simulink model "modele_non_lineaire"  (R2016a)
settings: Solver=ode45  StartTime=0.0  StopTime=tfin  FixedStep=0.001  RelTol=1e-09
undefined symbols (not defined in the file or in its folder): ae0, ae1, ae2, ae3, as0, as1, as2, as3, Axeq, Ayeq, be1, g, ia_e, ib_e, ic_e, JS, Jx, LA, mP, mS, Pzeq, RA, rS, vx_s_e, vy_s_e, vz_e, w_phi_e, w_theta_e, XA, XB, XC, XD, XE, XF, xSeq, YA, YB, YC, YD, YE, YF, ySeq
settings Model: Creator=delafontaine  LastModifiedBy=theh2203
settings SolverCC: AlgebraicLoopSolver=LineSearch
settings DataIOCC: LimitDataPoints=on  SaveFormat=Array  SignalLoggingSaveFormat=ModelDataLogs
settings DebuggingCC: UnderspecifiedInitializationDetection=Classic  MergeDetectMultiDrivingBlocksExec=none  MultiTaskDSMMsg=warning  MultiTaskCondExecSysMsg=none
settings HardwareCC: ProdBitPerPointer=32  ProdLargestAtomicFloat=None  ProdIntDivRoundTo=Undefined  ProdEndianess=Unspecified  ProdWordSize=32  ProdHWDeviceType=32-bit Generic
settings ModelReferenceCC: PropagateSignalLabelsOutOfModel=off
settings ConfigComp: CovModelRefEnable=Off  CovSFcnEnable=off

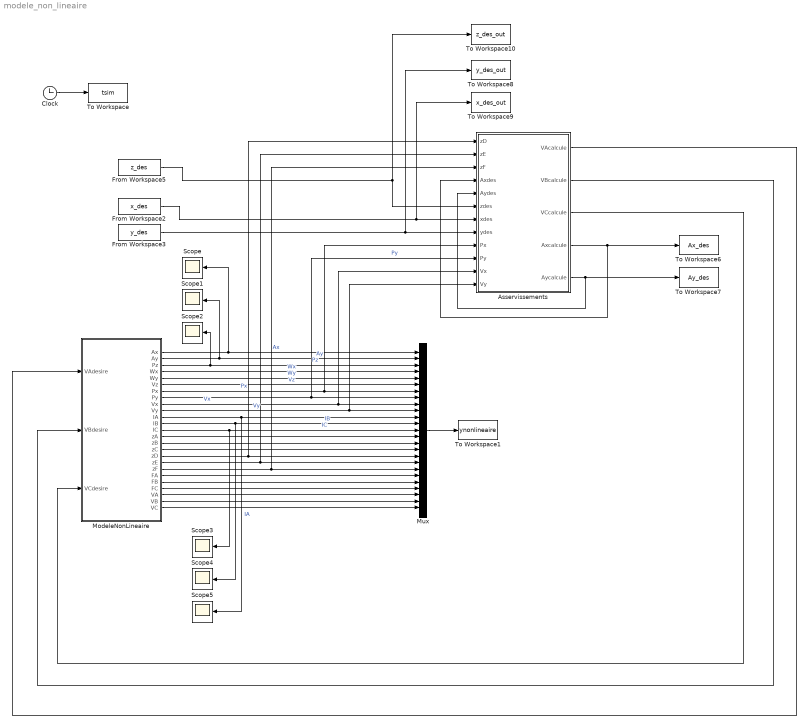
== system modele_non_lineaire ==
  Asservissements : Subsystem
      mask help: Simulink:masks:GenSFuncDesc_MD
      mask Help: eval('feval(''rtwprivate'',''rtwhelpview'',''rtw_sfcn_block'')');
  Clock : Clock
  From Workspace2 : FromWorkspace  VariableName=x_des  SampleTime=0  Interpolate=off  OutputAfterFinalValue=Holding final value
  From Workspace3 : FromWorkspace  VariableName=y_des  SampleTime=0  Interpolate=off  OutputAfterFinalValue=Holding final value
  From Workspace5 : FromWorkspace  VariableName=z_des  SampleTime=0  Interpolate=off  OutputAfterFinalValue=Holding final value
  ModeleNonLineaire : Subsystem
      mask help: Simulink:masks:GenSFuncDesc_MD
      mask Help: eval('feval(''rtwprivate'',''rtwhelpview'',''rtw_sfcn_block'')');
  Mux : Mux  Inputs=25
  Scope{,1..5} (6 alike) : Scope
  To Workspace : ToWorkspace  VariableName=tsim  SampleTime=-1
  To Workspace1 : ToWorkspace  VariableName=ynonlineaire  SampleTime=-1
  To Workspace10 : ToWorkspace  VariableName=z_des_out  SampleTime=-1
  To Workspace6 : ToWorkspace  VariableName=Ax_des  SampleTime=-1
  To Workspace7 : ToWorkspace  VariableName=Ay_des  SampleTime=-1
  To Workspace8 : ToWorkspace  VariableName=y_des_out  SampleTime=-1
  To Workspace9 : ToWorkspace  VariableName=x_des_out  SampleTime=-1
  wires:
  Mux/1 -> To Workspace1/1
  Clock/1 -> To Workspace/1
  From Workspace5/1 -> Asservissements/6(zdes), To Workspace10/1
  ModeleNonLineaire/1(Ax) -> Scope/1, Mux/1  "Ax"
  ModeleNonLineaire/2(Ay) -> Scope1/1, Mux/2  "Ay"
  ModeleNonLineaire/3(Pz) -> Scope2/1, Mux/3  "Pz"
  ModeleNonLineaire/4(Wx) -> Mux/4  "Wx"
  ModeleNonLineaire/5(Wy) -> Mux/5  "Wy"
  ModeleNonLineaire/6(Vz) -> Mux/6  "Vz"
  ModeleNonLineaire/7(Px) -> Asservissements/9(Px), Mux/7  "Px"
  ModeleNonLineaire/8(Py) -> Asservissements/10(Py), Mux/8  "Py"
  ModeleNonLineaire/9(Vx) -> Asservissements/11(Vx), Mux/9  "Vx"
  ModeleNonLineaire/10(Vy) -> Asservissements/12(Vy), Mux/10  "Vy"
  ModeleNonLineaire/11(IA) -> Scope5/1, Mux/11  "IA"
  ModeleNonLineaire/12(IB) -> Scope4/1, Mux/12  "IB"
  ModeleNonLineaire/13(IC) -> Scope3/1, Mux/13  "IC"
  From Workspace3/1 -> Asservissements/8(ydes), To Workspace8/1
  From Workspace2/1 -> Asservissements/7(xdes), To Workspace9/1
  ModeleNonLineaire/20(FA) -> Mux/20
  ModeleNonLineaire/21(FB) -> Mux/21
  ModeleNonLineaire/22(FC) -> Mux/22
  ModeleNonLineaire/23(VA) -> Mux/23
  ModeleNonLineaire/24(VB) -> Mux/24
  ModeleNonLineaire/25(VC) -> Mux/25
  ModeleNonLineaire/17(zD) -> Asservissements/1(zD), Mux/17
  ModeleNonLineaire/18(zE) -> Mux/18, Asservissements/2(zE)
  ModeleNonLineaire/19(zF) -> Asservissements/3(zF), Mux/19
  ModeleNonLineaire/14(zA) -> Mux/14
  ModeleNonLineaire/16(zC) -> Mux/16
  Asservissements/4(Axcalcule) -> Asservissements/4(Axdes), To Workspace6/1
  Asservissements/5(Aycalcule) -> Asservissements/5(Aydes), To Workspace7/1
  Asservissements/1(VAcalcule) -> ModeleNonLineaire/1(VAdesire)
  Asservissements/2(VBcalcule) -> ModeleNonLineaire/2(VBdesire)
  Asservissements/3(VCcalcule) -> ModeleNonLineaire/3(VCdesire)
  ModeleNonLineaire/15(zB) -> Mux/15

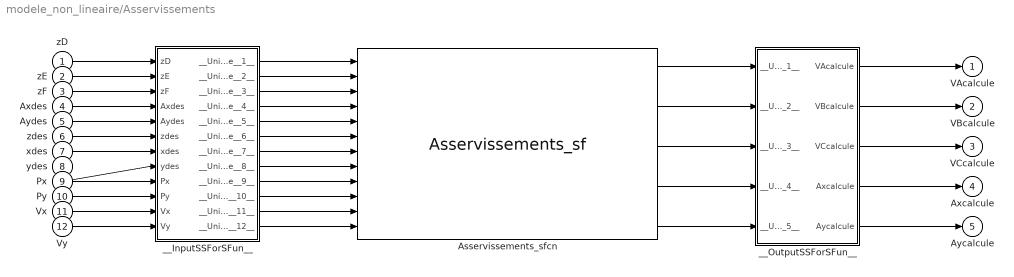
== system modele_non_lineaire/Asservissements ==
  zD : Inport
  zE : Inport  Port=2
  zF : Inport  Port=3
  Axdes : Inport  Port=4
  Aydes : Inport  Port=5
  zdes : Inport  Port=6
  xdes : Inport  Port=7
  ydes : Inport  Port=8
  Px : Inport  Port=9
  Py : Inport  Port=10
  Vx : Inport  Port=11
  Vy : Inport  Port=12
  Asservissements_sfcn : S-Function  FunctionName=Asservissements_sf  SFunctionModules=""  SFunctionDeploymentMode=off  EnableBusSupport=off  mask{rtw_sf_name=Asservissements_sf, showVar=off}
      mask prompts: rtw_sf_name "Simulink:masks:GenSFuncName_MP"; showVar "Simulink:masks:GenSFuncShowModuleList_MP"
      mask help: Simulink:masks:GenSFuncDesc_MD
      mask init:
      | displist = '';
      | if ~strcmp(get_param(gcb, 'FunctionName'), rtw_sf_name);
      |   set_param(gcb, 'FunctionName', rtw_sf_name);
      | end
      | % Check if we are generating code
      | rtw_mode = false;
      | if strcmpi(get_param(bdroot(gcb),'SimulationStatus'),'Initializing')
      | 	rtw_mode = strcmpi(get_param(bdroot(gcb),'BuildingRTWCode'),'on') && ...
      | 		~strcmpi(get_param(bdroot(gcb),'TargetStyle'),'SimulationTarget');
      | end
      | if showVar || rtw_mode
      | 	if exist('rtwsfunc') == 2 | exist('rtwsfunc') == 6
      | 		tmplist = rtwsfunc(rtw_sf_name,gcb);
      | 		tmplist = DAStudio.message('Simulink:masks:GenSFuncListOfModules_IC', tmplist);
      | 	elseif showVar
      | 		tmplist1 = DAStudio.message('Simulink:masks:GenSFuncListOfModules_IC', '');
      |         tmplist2 = DAStudio.message('Simulink:masks:GenSFuncNotLicensed_IC');
      |         tmplist = [tmplist1 tmplist2];
      |  	end
      | end
      | if showVar
      |   displist = tmplist;
      | end
      settings: CopyFcn=|
      | if ~strcmp(get_param(gcb,'Linkstatus'),'none') && ...
      | ~strcmp(get_param(gcb,'Linkstatus'),'implicit')
      |   set_param(gcb,'LinkStatus','none');
      | end
      mask Help: eval('feval(''rtwprivate'',''rtwhelpview'',''rtw_sfcn_block'')');
      mask Display:
      | port_label('input',1,'zD');
      | port_label('input',2,'zE');
      | port_label('input',3,'zF');
      | port_label('input',4,'Axdes');
      | port_label('input',5,'Aydes');
      | port_label('input',6,'zdes');
      | port_label('input',7,'xdes');
      | port_label('input',8,'ydes');
      | port_label('input',9,'Px');
      | port_label('input',10,'Py');
      | port_label('input',11,'Vx');
      | port_label('input',12,'Vy');
      | port_label('output',1,'VAcalcule');
      | port_label('output',2,'VBcalcule');
      | port_label('output',3,'VCcalcule');
      | port_label('output',4,'Axcalcule');
      | port_label('output',5,'Aycalcule');
  __InputSSForSFun__ : Subsystem
  __OutputSSForSFun__ : Subsystem
  VAcalcule : Outport
  VBcalcule : Outport  Port=2
  VCcalcule : Outport  Port=3
  Axcalcule : Outport  Port=4
  Aycalcule : Outport  Port=5
  wires:
  zD/1 -> __InputSSForSFun__/1(zD)
  zE/1 -> __InputSSForSFun__/2(zE)
  zF/1 -> __InputSSForSFun__/3(zF)
  Axdes/1 -> __InputSSForSFun__/4(Axdes)
  Aydes/1 -> __InputSSForSFun__/5(Aydes)
  zdes/1 -> __InputSSForSFun__/6(zdes)
  xdes/1 -> __InputSSForSFun__/7(xdes)
  ydes/1 -> __InputSSForSFun__/8(ydes)
  Px/1 -> __InputSSForSFun__/9(Px)
  Py/1 -> __InputSSForSFun__/10(Py)
  Vx/1 -> __InputSSForSFun__/11(Vx)
  Vy/1 -> __InputSSForSFun__/12(Vy)
  __InputSSForSFun__/1(__UniqueOutportName__1__) -> Asservissements_sfcn/1
  __InputSSForSFun__/2(__UniqueOutportName__2__) -> Asservissements_sfcn/2
  __InputSSForSFun__/3(__UniqueOutportName__3__) -> Asservissements_sfcn/3
  __InputSSForSFun__/4(__UniqueOutportName__4__) -> Asservissements_sfcn/4
  __InputSSForSFun__/5(__UniqueOutportName__5__) -> Asservissements_sfcn/5
  __InputSSForSFun__/6(__UniqueOutportName__6__) -> Asservissements_sfcn/6
  __InputSSForSFun__/7(__UniqueOutportName__7__) -> Asservissements_sfcn/7
  __InputSSForSFun__/8(__UniqueOutportName__8__) -> Asservissements_sfcn/8
  __InputSSForSFun__/9(__UniqueOutportName__9__) -> Asservissements_sfcn/9
  __InputSSForSFun__/10(__UniqueOutportName__10__) -> Asservissements_sfcn/10
  __InputSSForSFun__/11(__UniqueOutportName__11__) -> Asservissements_sfcn/11
  __InputSSForSFun__/12(__UniqueOutportName__12__) -> Asservissements_sfcn/12
  Asservissements_sfcn/1 -> __OutputSSForSFun__/1(__UniqueInportName__1__)
  Asservissements_sfcn/2 -> __OutputSSForSFun__/2(__UniqueInportName__2__)
  Asservissements_sfcn/3 -> __OutputSSForSFun__/3(__UniqueInportName__3__)
  Asservissements_sfcn/4 -> __OutputSSForSFun__/4(__UniqueInportName__4__)
  Asservissements_sfcn/5 -> __OutputSSForSFun__/5(__UniqueInportName__5__)
  __OutputSSForSFun__/1(VAcalcule) -> VAcalcule/1
  __OutputSSForSFun__/2(VBcalcule) -> VBcalcule/1
  __OutputSSForSFun__/3(VCcalcule) -> VCcalcule/1
  __OutputSSForSFun__/4(Axcalcule) -> Axcalcule/1
  __OutputSSForSFun__/5(Aycalcule) -> Aycalcule/1

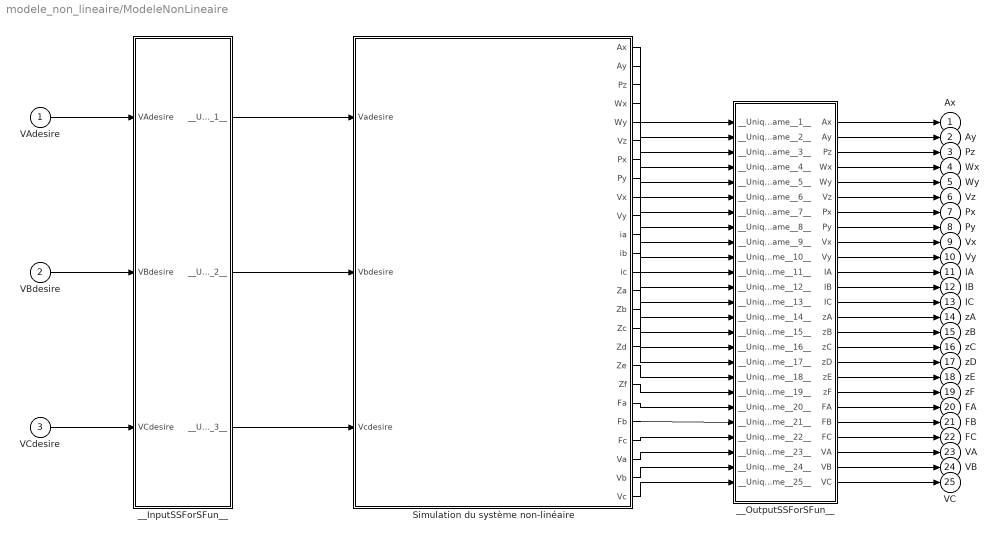
== system modele_non_lineaire/ModeleNonLineaire ==
  VAdesire : Inport
  VBdesire : Inport  Port=2
  VCdesire : Inport  Port=3
  Simulation du système non-linéaire : Subsystem
  __InputSSForSFun__ : Subsystem
  __OutputSSForSFun__ : Subsystem
  Ax : Outport
  Ay : Outport  Port=2
  Pz : Outport  Port=3
  Wx : Outport  Port=4
  Wy : Outport  Port=5
  Vz : Outport  Port=6
  Px : Outport  Port=7
  Py : Outport  Port=8
  Vx : Outport  Port=9
  Vy : Outport  Port=10
  IA : Outport  Port=11
  IB : Outport  Port=12
  IC : Outport  Port=13
  zA : Outport  Port=14
  zB : Outport  Port=15
  zC : Outport  Port=16
  zD : Outport  Port=17
  zE : Outport  Port=18
  zF : Outport  Port=19
  FA : Outport  Port=20
  FB : Outport  Port=21
  FC : Outport  Port=22
  VA : Outport  Port=23
  VB : Outport  Port=24
  VC : Outport  Port=25
  wires:
  VAdesire/1 -> __InputSSForSFun__/1(VAdesire)
  VBdesire/1 -> __InputSSForSFun__/2(VBdesire)
  VCdesire/1 -> __InputSSForSFun__/3(VCdesire)
  __InputSSForSFun__/1(__UniqueOutportName__1__) -> Simulation du système non-linéaire/1(Vadesire)
  __InputSSForSFun__/2(__UniqueOutportName__2__) -> Simulation du système non-linéaire/2(Vbdesire)
  __InputSSForSFun__/3(__UniqueOutportName__3__) -> Simulation du système non-linéaire/3(Vcdesire)
  Simulation du système non-linéaire/1(Ax) -> __OutputSSForSFun__/1(__UniqueInportName__1__)
  Simulation du système non-linéaire/2(Ay) -> __OutputSSForSFun__/2(__UniqueInportName__2__)
  Simulation du système non-linéaire/3(Pz) -> __OutputSSForSFun__/3(__UniqueInportName__3__)
  Simulation du système non-linéaire/4(Wx) -> __OutputSSForSFun__/4(__UniqueInportName__4__)
  Simulation du système non-linéaire/5(Wy) -> __OutputSSForSFun__/5(__UniqueInportName__5__)
  Simulation du système non-linéaire/6(Vz) -> __OutputSSForSFun__/6(__UniqueInportName__6__)
  Simulation du système non-linéaire/7(Px) -> __OutputSSForSFun__/7(__UniqueInportName__7__)
  Simulation du système non-linéaire/8(Py) -> __OutputSSForSFun__/8(__UniqueInportName__8__)
  Simulation du système non-linéaire/9(Vx) -> __OutputSSForSFun__/9(__UniqueInportName__9__)
  Simulation du système non-linéaire/10(Vy) -> __OutputSSForSFun__/10(__UniqueInportName__10__)
  Simulation du système non-linéaire/11(ia) -> __OutputSSForSFun__/11(__UniqueInportName__11__)
  Simulation du système non-linéaire/12(ib) -> __OutputSSForSFun__/12(__UniqueInportName__12__)
  Simulation du système non-linéaire/13(ic) -> __OutputSSForSFun__/13(__UniqueInportName__13__)
  Simulation du système non-linéaire/14(Za) -> __OutputSSForSFun__/14(__UniqueInportName__14__)
  Simulation du système non-linéaire/15(Zb) -> __OutputSSForSFun__/15(__UniqueInportName__15__)
  Simulation du système non-linéaire/16(Zc) -> __OutputSSForSFun__/16(__UniqueInportName__16__)
  Simulation du système non-linéaire/17(Zd) -> __OutputSSForSFun__/17(__UniqueInportName__17__)
  Simulation du système non-linéaire/18(Ze) -> __OutputSSForSFun__/18(__UniqueInportName__18__)
  Simulation du système non-linéaire/19(Zf) -> __OutputSSForSFun__/19(__UniqueInportName__19__)
  Simulation du système non-linéaire/20(Fa) -> __OutputSSForSFun__/20(__UniqueInportName__20__)
  Simulation du système non-linéaire/21(Fb) -> __OutputSSForSFun__/21(__UniqueInportName__21__)
  Simulation du système non-linéaire/22(Fc) -> __OutputSSForSFun__/22(__UniqueInportName__22__)
  Simulation du système non-linéaire/23(Va) -> __OutputSSForSFun__/23(__UniqueInportName__23__)
  Simulation du système non-linéaire/24(Vb) -> __OutputSSForSFun__/24(__UniqueInportName__24__)
  Simulation du système non-linéaire/25(Vc) -> __OutputSSForSFun__/25(__UniqueInportName__25__)
  __OutputSSForSFun__/1(Ax) -> Ax/1
  __OutputSSForSFun__/2(Ay) -> Ay/1
  __OutputSSForSFun__/3(Pz) -> Pz/1
  __OutputSSForSFun__/4(Wx) -> Wx/1
  __OutputSSForSFun__/5(Wy) -> Wy/1
  __OutputSSForSFun__/6(Vz) -> Vz/1
  __OutputSSForSFun__/7(Px) -> Px/1
  __OutputSSForSFun__/8(Py) -> Py/1
  __OutputSSForSFun__/9(Vx) -> Vx/1
  __OutputSSForSFun__/10(Vy) -> Vy/1
  __OutputSSForSFun__/11(IA) -> IA/1
  __OutputSSForSFun__/12(IB) -> IB/1
  __OutputSSForSFun__/13(IC) -> IC/1
  __OutputSSForSFun__/14(zA) -> zA/1
  __OutputSSForSFun__/15(zB) -> zB/1
  __OutputSSForSFun__/16(zC) -> zC/1
  __OutputSSForSFun__/17(zD) -> zD/1
  __OutputSSForSFun__/18(zE) -> zE/1
  __OutputSSForSFun__/19(zF) -> zF/1
  __OutputSSForSFun__/20(FA) -> FA/1
  __OutputSSForSFun__/21(FB) -> FB/1
  __OutputSSForSFun__/22(FC) -> FC/1
  __OutputSSForSFun__/23(VA) -> VA/1
  __OutputSSForSFun__/24(VB) -> VB/1
  __OutputSSForSFun__/25(VC) -> VC/1

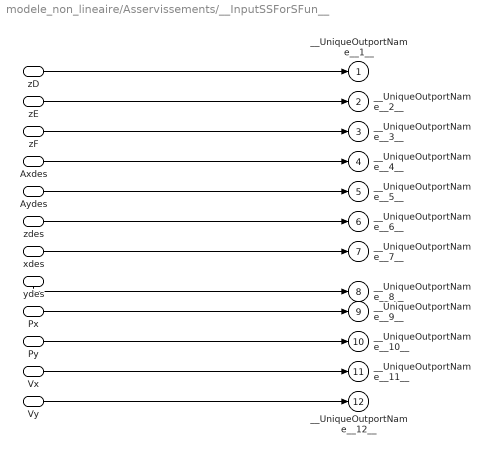
== system modele_non_lineaire/Asservissements/__InputSSForSFun__ ==
  zD : Inport
  zE : Inport  Port=2
  zF : Inport  Port=3
  Axdes : Inport  Port=4
  Aydes : Inport  Port=5
  zdes : Inport  Port=6
  xdes : Inport  Port=7
  ydes : Inport  Port=8
  Px : Inport  Port=9
  Py : Inport  Port=10
  Vx : Inport  Port=11
  Vy : Inport  Port=12
  __UniqueOutportName__1__ : Outport
  __UniqueOutportName__2__ : Outport  Port=2
  __UniqueOutportName__3__ : Outport  Port=3
  __UniqueOutportName__4__ : Outport  Port=4
  __UniqueOutportName__5__ : Outport  Port=5
  __UniqueOutportName__6__ : Outport  Port=6
  __UniqueOutportName__7__ : Outport  Port=7
  __UniqueOutportName__8__ : Outport  Port=8
  __UniqueOutportName__9__ : Outport  Port=9
  __UniqueOutportName__10__ : Outport  Port=10
  __UniqueOutportName__11__ : Outport  Port=11
  __UniqueOutportName__12__ : Outport  Port=12
  wires:
  zD/1 -> __UniqueOutportName__1__/1
  zE/1 -> __UniqueOutportName__2__/1
  zF/1 -> __UniqueOutportName__3__/1
  Axdes/1 -> __UniqueOutportName__4__/1
  Aydes/1 -> __UniqueOutportName__5__/1
  zdes/1 -> __UniqueOutportName__6__/1
  xdes/1 -> __UniqueOutportName__7__/1
  ydes/1 -> __UniqueOutportName__8__/1
  Px/1 -> __UniqueOutportName__9__/1
  Py/1 -> __UniqueOutportName__10__/1
  Vx/1 -> __UniqueOutportName__11__/1
  Vy/1 -> __UniqueOutportName__12__/1

== system modele_non_lineaire/Asservissements/__OutputSSForSFun__ ==
  __UniqueInportName__1__ : Inport
  __UniqueInportName__2__ : Inport  Port=2
  __UniqueInportName__3__ : Inport  Port=3
  __UniqueInportName__4__ : Inport  Port=4
  __UniqueInportName__5__ : Inport  Port=5
  VAcalcule : Outport
  VBcalcule : Outport  Port=2
  VCcalcule : Outport  Port=3
  Axcalcule : Outport  Port=4
  Aycalcule : Outport  Port=5
  wires:
  __UniqueInportName__1__/1 -> VAcalcule/1
  __UniqueInportName__2__/1 -> VBcalcule/1
  __UniqueInportName__3__/1 -> VCcalcule/1
  __UniqueInportName__4__/1 -> Axcalcule/1  "Ax_des"
  __UniqueInportName__5__/1 -> Aycalcule/1  "Ay_des"

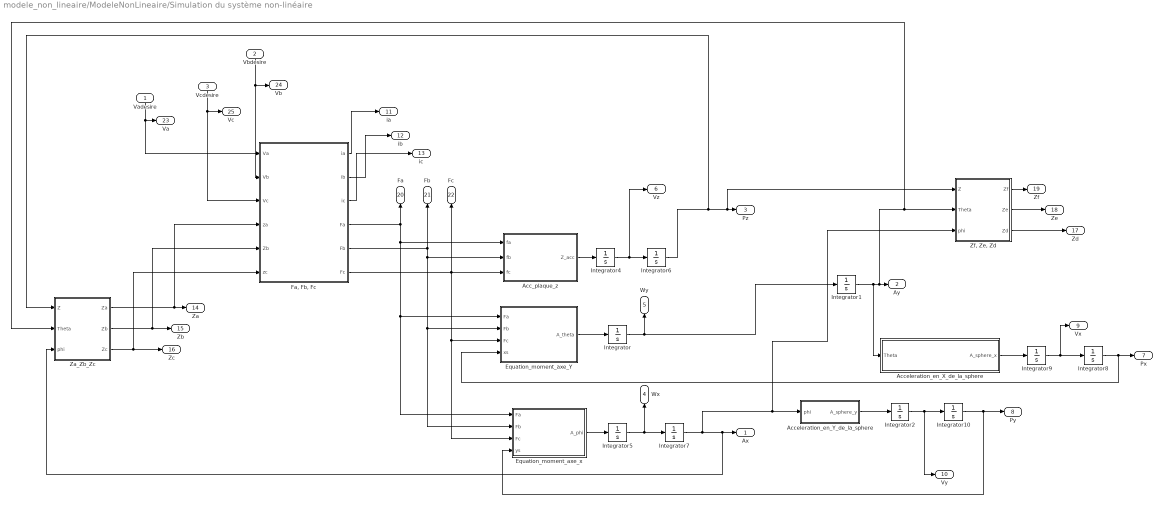
== system modele_non_lineaire/ModeleNonLineaire/Simulation du système non-linéaire ==
  Vadesire : Inport
  Vbdesire : Inport  Port=2
  Vcdesire : Inport  Port=3
  Acc_plaque_z : Subsystem
  Acceleration_en_X_de_la_sphere : Subsystem
  Acceleration_en_Y_de_la_sphere : Subsystem
  Equation_moment_axe_Y : Subsystem
  Equation_moment_axe_x : Subsystem
  "Fa, Fb, Fc" : Subsystem
  Integrator : Integrator  InitialCondition=w_theta_e
  Integrator1 : Integrator  InitialCondition=Ayeq
  Integrator10 : Integrator  InitialCondition=ySeq
  Integrator2 : Integrator  InitialCondition=vy_s_e
  Integrator4 : Integrator  InitialCondition=vz_e
  Integrator5 : Integrator  InitialCondition=w_phi_e
  Integrator6 : Integrator  InitialCondition=Pzeq
  Integrator7 : Integrator  InitialCondition=Axeq
  Integrator8 : Integrator  InitialCondition=xSeq
  Integrator9 : Integrator  InitialCondition=vx_s_e
  Za_Zb_Zc : Subsystem
  "Zf, Ze, Zd" : Subsystem
  Ax : Outport
  Ay : Outport  Port=2
  Pz : Outport  Port=3
  Wx : Outport  Port=4
  Wy : Outport  Port=5
  Vz : Outport  Port=6
  Px : Outport  Port=7
  Py : Outport  Port=8
  Vx : Outport  Port=9
  Vy : Outport  Port=10
  ia : Outport  Port=11
  ib : Outport  Port=12
  ic : Outport  Port=13
  Za : Outport  Port=14
  Zb : Outport  Port=15
  Zc : Outport  Port=16
  Zd : Outport  Port=17
  Ze : Outport  Port=18
  Zf : Outport  Port=19
  Fa : Outport  Port=20
  Fb : Outport  Port=21
  Fc : Outport  Port=22
  Va : Outport  Port=23
  Vb : Outport  Port=24
  Vc : Outport  Port=25
  wires:
  Vadesire/1 -> "Fa, Fb, Fc"/1(Va), Va/1
  "Fa, Fb, Fc"/3(ic) -> ic/1
  "Fa, Fb, Fc"/1(ia) -> ia/1
  "Fa, Fb, Fc"/2(ib) -> ib/1
  Vcdesire/1 -> "Fa, Fb, Fc"/3(Vc), Vc/1
  Vbdesire/1 -> Vb/1, "Fa, Fb, Fc"/2(Vb)
  "Zf, Ze, Zd"/1(Zf) -> Zf/1
  "Zf, Ze, Zd"/2(Ze) -> Ze/1
  "Zf, Ze, Zd"/3(Zd) -> Zd/1
  Integrator/1 -> Integrator1/1, Wy/1
  Integrator1/1 -> Acceleration_en_X_de_la_sphere/1(Theta), Za_Zb_Zc/2(Theta), "Zf, Ze, Zd"/2(Theta), Ay/1
  Integrator5/1 -> Integrator7/1, Wx/1
  Integrator7/1 -> "Zf, Ze, Zd"/3(phi), Acceleration_en_Y_de_la_sphere/1(phi), Za_Zb_Zc/3(phi), Ax/1
  Acc_plaque_z/1(Z_acc) -> Integrator4/1
  Integrator4/1 -> Vz/1, Integrator6/1
  Integrator6/1 -> Za_Zb_Zc/1(Z), "Zf, Ze, Zd"/1(Z), Pz/1
  Acceleration_en_X_de_la_sphere/1(A_sphere_x) -> Integrator9/1
  Integrator9/1 -> Vx/1, Integrator8/1
  Integrator8/1 -> Equation_moment_axe_Y/4(xs), Px/1
  Integrator10/1 -> Equation_moment_axe_x/4(ys), Py/1
  Acceleration_en_Y_de_la_sphere/1(A_sphere_y) -> Integrator2/1
  Integrator2/1 -> Vy/1, Integrator10/1
  Za_Zb_Zc/1(Za) -> "Fa, Fb, Fc"/4(za), Za/1
  Za_Zb_Zc/2("Zb ") -> "Fa, Fb, Fc"/5(Zb), Zb/1
  Za_Zb_Zc/3(Zc) -> "Fa, Fb, Fc"/6(zc), Zc/1
  Equation_moment_axe_x/1(A_phi) -> Integrator5/1
  Equation_moment_axe_Y/1(A_theta) -> Integrator/1
  "Fa, Fb, Fc"/4(Fa) -> Fa/1, Equation_moment_axe_x/1(Fa), Equation_moment_axe_Y/1(Fa), Acc_plaque_z/1(fa)
  "Fa, Fb, Fc"/5(Fb) -> Fb/1, Equation_moment_axe_x/2(Fb), Equation_moment_axe_Y/2(Fb), Acc_plaque_z/2(fb)
  "Fa, Fb, Fc"/6(Fc) -> Equation_moment_axe_x/3(Fc), Equation_moment_axe_Y/3(Fc), Fc/1, Acc_plaque_z/3(fc)

== system modele_non_lineaire/ModeleNonLineaire/__InputSSForSFun__ ==
  VAdesire : Inport
  VBdesire : Inport  Port=2
  VCdesire : Inport  Port=3
  __UniqueOutportName__1__ : Outport
  __UniqueOutportName__2__ : Outport  Port=2
  __UniqueOutportName__3__ : Outport  Port=3
  wires:
  VAdesire/1 -> __UniqueOutportName__1__/1
  VBdesire/1 -> __UniqueOutportName__2__/1
  VCdesire/1 -> __UniqueOutportName__3__/1

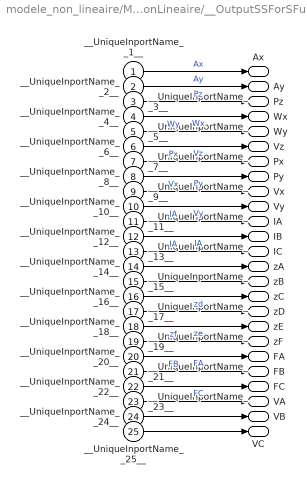
== system modele_non_lineaire/ModeleNonLineaire/__OutputSSForSFun__ ==
  __UniqueInportName__1__ : Inport
  __UniqueInportName__2__ : Inport  Port=2
  __UniqueInportName__3__ : Inport  Port=3
  __UniqueInportName__4__ : Inport  Port=4
  __UniqueInportName__5__ : Inport  Port=5
  __UniqueInportName__6__ : Inport  Port=6
  __UniqueInportName__7__ : Inport  Port=7
  __UniqueInportName__8__ : Inport  Port=8
  __UniqueInportName__9__ : Inport  Port=9
  __UniqueInportName__10__ : Inport  Port=10
  __UniqueInportName__11__ : Inport  Port=11
  __UniqueInportName__12__ : Inport  Port=12
  __UniqueInportName__13__ : Inport  Port=13
  __UniqueInportName__14__ : Inport  Port=14
  __UniqueInportName__15__ : Inport  Port=15
  __UniqueInportName__16__ : Inport  Port=16
  __UniqueInportName__17__ : Inport  Port=17
  __UniqueInportName__18__ : Inport  Port=18
  __UniqueInportName__19__ : Inport  Port=19
  __UniqueInportName__20__ : Inport  Port=20
  __UniqueInportName__21__ : Inport  Port=21
  __UniqueInportName__22__ : Inport  Port=22
  __UniqueInportName__23__ : Inport  Port=23
  __UniqueInportName__24__ : Inport  Port=24
  __UniqueInportName__25__ : Inport  Port=25
  Ax : Outport
  Ay : Outport  Port=2
  Pz : Outport  Port=3
  Wx : Outport  Port=4
  Wy : Outport  Port=5
  Vz : Outport  Port=6
  Px : Outport  Port=7
  Py : Outport  Port=8
  Vx : Outport  Port=9
  Vy : Outport  Port=10
  IA : Outport  Port=11
  IB : Outport  Port=12
  IC : Outport  Port=13
  zA : Outport  Port=14
  zB : Outport  Port=15
  zC : Outport  Port=16
  zD : Outport  Port=17
  zE : Outport  Port=18
  zF : Outport  Port=19
  FA : Outport  Port=20
  FB : Outport  Port=21
  FC : Outport  Port=22
  VA : Outport  Port=23
  VB : Outport  Port=24
  VC : Outport  Port=25
  wires:
  __UniqueInportName__1__/1 -> Ax/1  "Ax"
  __UniqueInportName__2__/1 -> Ay/1  "Ay"
  __UniqueInportName__3__/1 -> Pz/1  "Pz"
  __UniqueInportName__4__/1 -> Wx/1  "Wx"
  __UniqueInportName__5__/1 -> Wy/1  "Wy"
  __UniqueInportName__6__/1 -> Vz/1  "Vz"
  __UniqueInportName__7__/1 -> Px/1  "Px"
  __UniqueInportName__8__/1 -> Py/1  "Py"
  __UniqueInportName__9__/1 -> Vx/1  "Vx"
  __UniqueInportName__10__/1 -> Vy/1  "Vy"
  __UniqueInportName__11__/1 -> IA/1  "IA"
  __UniqueInportName__12__/1 -> IB/1  "IA"
  __UniqueInportName__13__/1 -> IC/1  "IA"
  __UniqueInportName__14__/1 -> zA/1
  __UniqueInportName__15__/1 -> zB/1
  __UniqueInportName__16__/1 -> zC/1
  __UniqueInportName__17__/1 -> zD/1  "zd"
  __UniqueInportName__18__/1 -> zE/1  "ze"
  __UniqueInportName__19__/1 -> zF/1  "zf"
  __UniqueInportName__20__/1 -> FA/1  "FA"
  __UniqueInportName__21__/1 -> FB/1  "FB"
  __UniqueInportName__22__/1 -> FC/1  "FC"
  __UniqueInportName__23__/1 -> VA/1
  __UniqueInportName__24__/1 -> VB/1
  __UniqueInportName__25__/1 -> VC/1

== system modele_non_lineaire/ModeleNonLineaire/Simulation du système non-linéaire/Acc_plaque_z ==
  fa : Inport
  fb : Inport  Port=2
  fc : Inport  Port=3
  Add : Sum  Inputs=++++
  Divide : Product  Inputs=*/
  Gain : Gain  Gain=g
  "masse_plaque-sphere " : Constant  Value=mP+mS
  Z_acc : Outport
  wires:
  fa/1 -> Add/1
  fc/1 -> Add/3
  fb/1 -> Add/2
  Add/1 -> Divide/1
  Divide/1 -> Z_acc/1
  "masse_plaque-sphere "/1 -> Divide/2, Gain/1
  Gain/1 -> Add/4

== system modele_non_lineaire/ModeleNonLineaire/Simulation du système non-linéaire/Acceleration_en_X_de_la_sphere ==
  Theta : Inport
  Add : Sum
  Constant : Constant  Value=mS
  Constant1 : Constant  Value=JS/rS^2
  Divide : Product  Inputs=*/
  Gain : Gain  Gain=-g*mS
  A_sphere_x : Outport
  wires:
  Theta/1 -> Gain/1
  Gain/1 -> Divide/1
  Constant1/1 -> Add/2
  Constant/1 -> Add/1
  Add/1 -> Divide/2
  Divide/1 -> A_sphere_x/1

== system modele_non_lineaire/ModeleNonLineaire/Simulation du système non-linéaire/Acceleration_en_Y_de_la_sphere ==
  phi : Inport
  Add : Sum
  Constant : Constant  Value=mS
  Constant1 : Constant  Value=JS/rS^2
  Divide : Product  Inputs=*/
  Gain : Gain  Gain=g*mS
  A_sphere_y : Outport
  wires:
  phi/1 -> Gain/1
  Gain/1 -> Divide/1
  Constant1/1 -> Add/2
  Constant/1 -> Add/1
  Add/1 -> Divide/2
  Divide/1 -> A_sphere_y/1

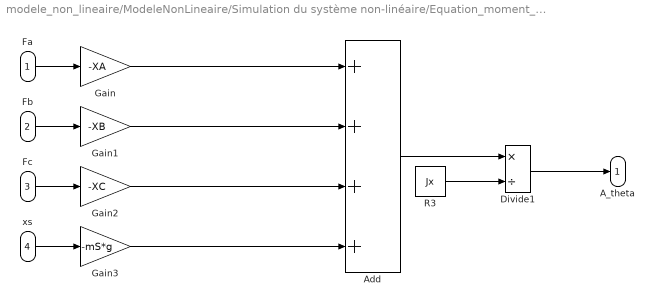
== system modele_non_lineaire/ModeleNonLineaire/Simulation du système non-linéaire/Equation_moment_axe_Y ==
  Fa : Inport
  Fb : Inport  Port=2
  Fc : Inport  Port=3
  xs : Inport  Port=4
  Add : Sum  Inputs=++++
  Divide1 : Product  Inputs=*/
  Gain : Gain  Gain=-XA
  Gain1 : Gain  Gain=-XB
  Gain2 : Gain  Gain=-XC
  Gain3 : Gain  Gain=-mS*g
  R3 : Constant  Value=Jx
  A_theta : Outport
  wires:
  Add/1 -> Divide1/1
  Divide1/1 -> A_theta/1
  Fa/1 -> Gain/1
  Gain/1 -> Add/1
  Fb/1 -> Gain1/1
  Fc/1 -> Gain2/1
  Gain2/1 -> Add/3
  Gain1/1 -> Add/2
  xs/1 -> Gain3/1
  R3/1 -> Divide1/2
  Gain3/1 -> Add/4

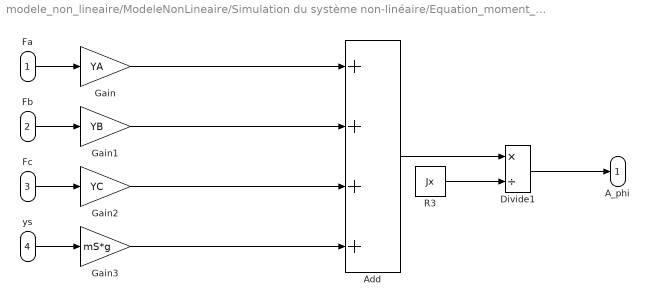
== system modele_non_lineaire/ModeleNonLineaire/Simulation du système non-linéaire/Equation_moment_axe_x ==
  Fa : Inport
  Fb : Inport  Port=2
  Fc : Inport  Port=3
  ys : Inport  Port=4
  Add : Sum  Inputs=++++
  Divide1 : Product  Inputs=*/
  Gain : Gain  Gain=YA
  Gain1 : Gain  Gain=YB
  Gain2 : Gain  Gain=YC
  Gain3 : Gain  Gain=mS*g
  R3 : Constant  Value=Jx
  A_phi : Outport
  wires:
  Gain3/1 -> Add/4
  R3/1 -> Divide1/2
  ys/1 -> Gain3/1
  Gain1/1 -> Add/2
  Gain2/1 -> Add/3
  Fc/1 -> Gain2/1
  Fb/1 -> Gain1/1
  Gain/1 -> Add/1
  Fa/1 -> Gain/1
  Divide1/1 -> A_phi/1
  Add/1 -> Divide1/1

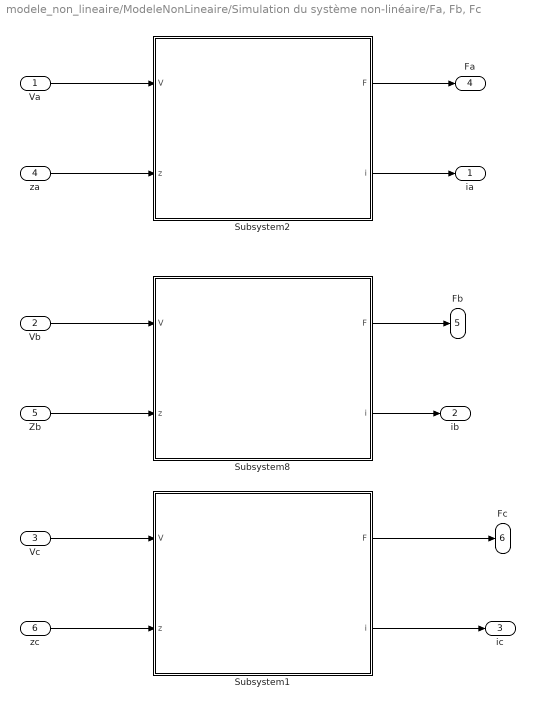
== system modele_non_lineaire/ModeleNonLineaire/Simulation du système non-linéaire/Fa, Fb, Fc ==
  Va : Inport
  Vb : Inport  Port=2
  Vc : Inport  Port=3
  za : Inport  Port=4
  Zb : Inport  Port=5
  zc : Inport  Port=6
  Subsystem1 : Subsystem
  Subsystem2 : Subsystem
  Subsystem8 : Subsystem
  ia : Outport
  ib : Outport  Port=2
  ic : Outport  Port=3
  Fa : Outport  Port=4
  Fb : Outport  Port=5
  Fc : Outport  Port=6
  wires:
  za/1 -> Subsystem2/2(z)
  Va/1 -> Subsystem2/1(V)
  Zb/1 -> Subsystem8/2(z)
  zc/1 -> Subsystem1/2(z)
  Subsystem1/1(F) -> Fc/1
  Subsystem8/1(F) -> Fb/1
  Vb/1 -> Subsystem8/1(V)
  Vc/1 -> Subsystem1/1(V)
  Subsystem2/1(F) -> Fa/1
  Subsystem2/2(i) -> ia/1
  Subsystem8/2(i) -> ib/1
  Subsystem1/2(i) -> ic/1

== system modele_non_lineaire/ModeleNonLineaire/Simulation du système non-linéaire/Za_Zb_Zc ==
  Z : Inport
  Theta : Inport  Port=2
  phi : Inport  Port=3
  pos_Za : Subsystem
  pos_Zb : Subsystem
  pos_Zc : Subsystem
  Za : Outport
  "Zb " : Outport  Port=2
  Zc : Outport  Port=3
  wires:
  pos_Zc/1("Zc ") -> Zc/1
  pos_Zb/1(Zb) -> "Zb "/1
  pos_Za/1(Za) -> Za/1
  Theta/1 -> pos_Za/1(theta), pos_Zc/1(theta), pos_Zb/1(theta)
  phi/1 -> pos_Za/2(phi), pos_Zc/2(phi), pos_Zb/2(phi)
  Z/1 -> pos_Za/3(Z), pos_Zc/3(Z), pos_Zb/3(Z)

== system modele_non_lineaire/ModeleNonLineaire/Simulation du système non-linéaire/Zf, Ze, Zd ==
  Z : Inport
  Theta : Inport  Port=2
  phi : Inport  Port=3
  pos_ZF : Subsystem
  pos_Zd : Subsystem
  pos_Ze : Subsystem
  Zf : Outport
  Ze : Outport  Port=2
  Zd : Outport  Port=3
  wires:
  pos_Zd/1(Zd) -> Zd/1
  pos_ZF/1(Zf) -> Zf/1
  pos_Ze/1(Ze) -> Ze/1
  Theta/1 -> pos_Ze/1(theta), pos_Zd/1(theta), pos_ZF/1(theta)
  phi/1 -> pos_Ze/2(phi), pos_Zd/2(phi), pos_ZF/2(phi)
  Z/1 -> pos_Ze/3(Z), pos_Zd/3(Z), pos_ZF/3(Z)

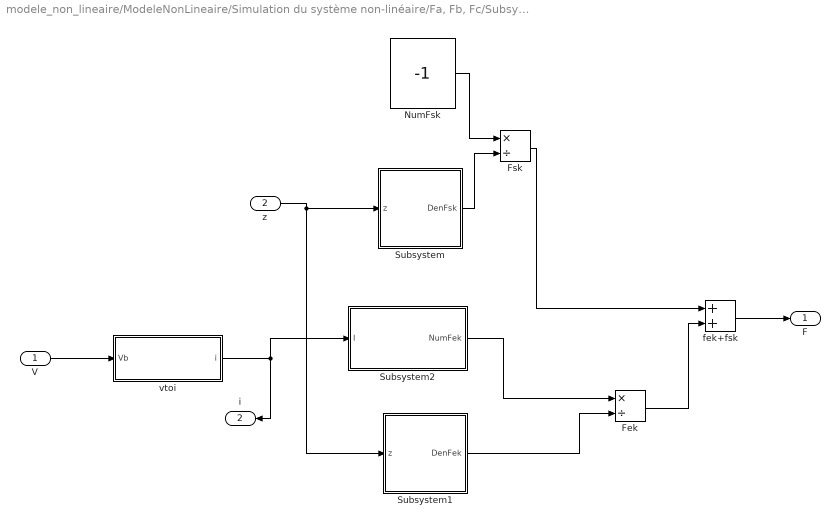
== system modele_non_lineaire/ModeleNonLineaire/Simulation du système non-linéaire/Fa, Fb, Fc/Subsystem1 ==
  V : Inport
  z : Inport  Port=2
  Fek : Product  Inputs=*/
  Fsk : Product  Inputs=*/
  NumFsk : Constant  Value=-1
  Subsystem : Subsystem
  Subsystem1 : Subsystem
  Subsystem2 : Subsystem
  fek+fsk : Sum
  vtoi : Subsystem
  F : Outport
  i : Outport  Port=2
  wires:
  fek+fsk/1 -> F/1
  NumFsk/1 -> Fsk/1
  Fsk/1 -> fek+fsk/1
  vtoi/1(i) -> i/1, Subsystem2/1(I)
  V/1 -> vtoi/1(Vb)
  z/1 -> Subsystem1/1(z), Subsystem/1(z)
  Subsystem/1(DenFsk) -> Fsk/2
  Subsystem1/1(DenFek) -> Fek/2
  Fek/1 -> fek+fsk/2
  Subsystem2/1(NumFek) -> Fek/1

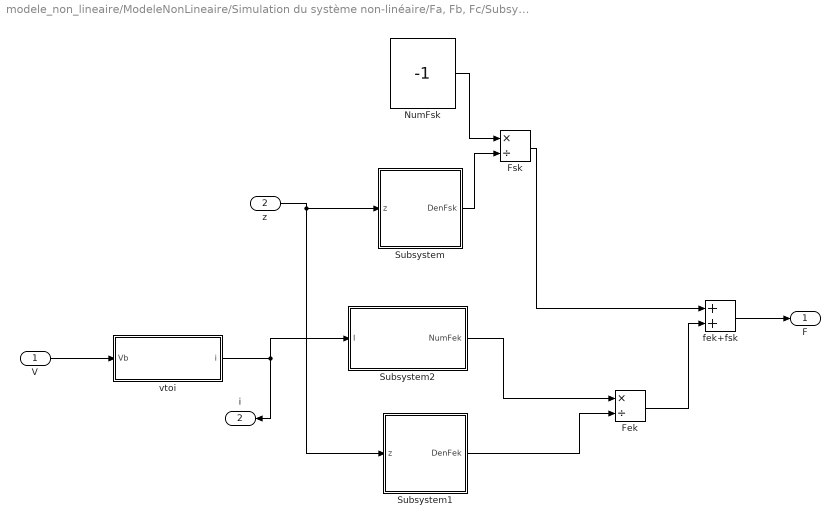
== system modele_non_lineaire/ModeleNonLineaire/Simulation du système non-linéaire/Fa, Fb, Fc/Subsystem2 ==
  V : Inport
  z : Inport  Port=2
  Fek : Product  Inputs=*/
  Fsk : Product  Inputs=*/
  NumFsk : Constant  Value=-1
  Subsystem : Subsystem
  Subsystem1 : Subsystem
  Subsystem2 : Subsystem
  fek+fsk : Sum
  vtoi : Subsystem
  F : Outport
  i : Outport  Port=2
  wires:
  fek+fsk/1 -> F/1
  NumFsk/1 -> Fsk/1
  Fsk/1 -> fek+fsk/1
  vtoi/1(i) -> i/1, Subsystem2/1(I)
  V/1 -> vtoi/1(Vb)
  z/1 -> Subsystem1/1(z), Subsystem/1(z)
  Subsystem/1(DenFsk) -> Fsk/2
  Subsystem1/1(DenFek) -> Fek/2
  Fek/1 -> fek+fsk/2
  Subsystem2/1(NumFek) -> Fek/1

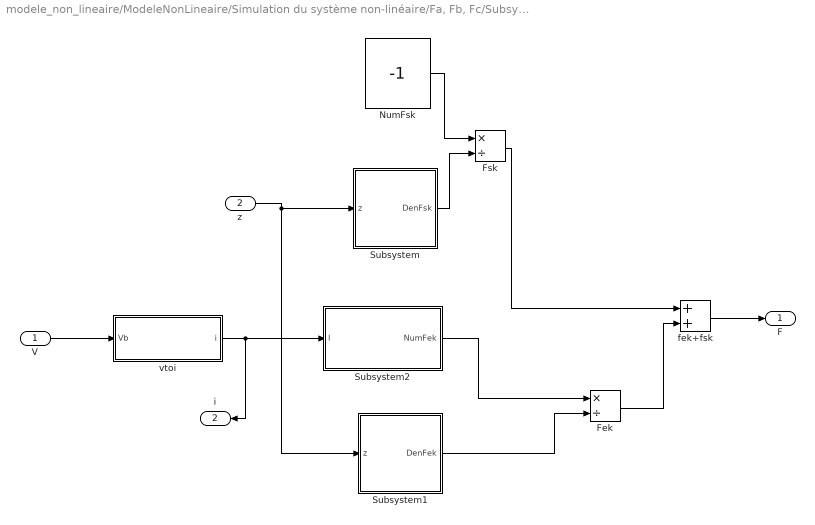
== system modele_non_lineaire/ModeleNonLineaire/Simulation du système non-linéaire/Fa, Fb, Fc/Subsystem8 ==
  V : Inport
  z : Inport  Port=2
  Fek : Product  Inputs=*/
  Fsk : Product  Inputs=*/
  NumFsk : Constant  Value=-1
  Subsystem : Subsystem
  Subsystem1 : Subsystem
  Subsystem2 : Subsystem
  fek+fsk : Sum
  vtoi : Subsystem
  F : Outport
  i : Outport  Port=2
  wires:
  fek+fsk/1 -> F/1
  NumFsk/1 -> Fsk/1
  Fsk/1 -> fek+fsk/1
  vtoi/1(i) -> i/1, Subsystem2/1(I)
  V/1 -> vtoi/1(Vb)
  z/1 -> Subsystem1/1(z), Subsystem/1(z)
  Subsystem/1(DenFsk) -> Fsk/2
  Subsystem1/1(DenFek) -> Fek/2
  Fek/1 -> fek+fsk/2
  Subsystem2/1(NumFek) -> Fek/1

== system modele_non_lineaire/ModeleNonLineaire/Simulation du système non-linéaire/Za_Zb_Zc/pos_Za ==
  theta : Inport
  phi : Inport  Port=2
  Z : Inport  Port=3
  Add : Sum  Inputs=+++
  Gain : Gain  Gain=YA
  Gain1 : Gain  Gain=-XA
  Za : Outport
  wires:
  phi/1 -> Gain/1
  theta/1 -> Gain1/1
  Gain/1 -> Add/1
  Gain1/1 -> Add/2
  Z/1 -> Add/3
  Add/1 -> Za/1

== system modele_non_lineaire/ModeleNonLineaire/Simulation du système non-linéaire/Za_Zb_Zc/pos_Zb ==
  theta : Inport
  phi : Inport  Port=2
  Z : Inport  Port=3
  Add : Sum  Inputs=+++
  Gain : Gain  Gain=YB
  Gain1 : Gain  Gain=-XB
  Zb : Outport
  wires:
  phi/1 -> Gain/1
  theta/1 -> Gain1/1
  Gain/1 -> Add/1
  Gain1/1 -> Add/2
  Z/1 -> Add/3
  Add/1 -> Zb/1

== system modele_non_lineaire/ModeleNonLineaire/Simulation du système non-linéaire/Za_Zb_Zc/pos_Zc ==
  theta : Inport
  phi : Inport  Port=2
  Z : Inport  Port=3
  Add : Sum  Inputs=+++
  Gain : Gain  Gain=YC
  Gain1 : Gain  Gain=-XC
  "Zc " : Outport
  wires:
  phi/1 -> Gain/1
  theta/1 -> Gain1/1
  Gain/1 -> Add/1
  Gain1/1 -> Add/2
  Z/1 -> Add/3
  Add/1 -> "Zc "/1

== system modele_non_lineaire/ModeleNonLineaire/Simulation du système non-linéaire/Zf, Ze, Zd/pos_ZF ==
  theta : Inport
  phi : Inport  Port=2
  Z : Inport  Port=3
  Add : Sum  Inputs=+++
  Gain : Gain  Gain=YF
  Gain1 : Gain  Gain=-XF
  Zf : Outport
  wires:
  phi/1 -> Gain/1
  theta/1 -> Gain1/1
  Gain/1 -> Add/1
  Gain1/1 -> Add/2
  Z/1 -> Add/3
  Add/1 -> Zf/1

== system modele_non_lineaire/ModeleNonLineaire/Simulation du système non-linéaire/Zf, Ze, Zd/pos_Zd ==
  theta : Inport
  phi : Inport  Port=2
  Z : Inport  Port=3
  Add : Sum  Inputs=+++
  Gain : Gain  Gain=YD
  Gain1 : Gain  Gain=-XD
  Zd : Outport
  wires:
  phi/1 -> Gain/1
  theta/1 -> Gain1/1
  Gain/1 -> Add/1
  Gain1/1 -> Add/2
  Z/1 -> Add/3
  Add/1 -> Zd/1

== system modele_non_lineaire/ModeleNonLineaire/Simulation du système non-linéaire/Zf, Ze, Zd/pos_Ze ==
  theta : Inport
  phi : Inport  Port=2
  Z : Inport  Port=3
  Add : Sum  Inputs=+++
  Gain : Gain  Gain=YE
  Gain1 : Gain  Gain=-XE
  Ze : Outport
  wires:
  phi/1 -> Gain/1
  theta/1 -> Gain1/1
  Gain/1 -> Add/1
  Gain1/1 -> Add/2
  Z/1 -> Add/3
  Add/1 -> Ze/1

== system modele_non_lineaire/ModeleNonLineaire/Simulation du système non-linéaire/Fa, Fb, Fc/Subsystem1/Subsystem ==
  z : Inport
  Add : Sum  Inputs=++++
  Constant : Constant  Value=as0
  Constant1 : Constant  Value=as1
  Constant2 : Constant  Value=as2
  Constant3 : Constant  Value=as3
  Product4 : Product
  Product5 : Product  Inputs=3
  Product6 : Product  Inputs=4
  DenFsk : Outport
  wires:
  Constant/1 -> Add/1
  Product5/1 -> Add/3
  Product4/1 -> Add/2
  Product6/1 -> Add/4
  z/1 -> Product5/3, Product6/1, Product6/4, Product6/3, Product5/1, Product4/1
  Constant1/1 -> Product4/2
  Constant2/1 -> Product5/2
  Constant3/1 -> Product6/2
  Add/1 -> DenFsk/1

== system modele_non_lineaire/ModeleNonLineaire/Simulation du système non-linéaire/Fa, Fb, Fc/Subsystem1/Subsystem1 ==
  z : Inport
  Add : Sum  Inputs=++++
  Constant : Constant  Value=ae0
  Constant1 : Constant  Value=ae1
  Constant2 : Constant  Value=ae2
  Constant3 : Constant  Value=ae3
  Product4 : Product
  Product5 : Product  Inputs=3
  Product6 : Product  Inputs=4
  DenFek : Outport
  wires:
  Constant/1 -> Add/1
  Product5/1 -> Add/3
  Product4/1 -> Add/2
  Product6/1 -> Add/4
  z/1 -> Product5/3, Product6/1, Product6/4, Product6/3, Product5/1, Product4/1
  Constant1/1 -> Product4/2
  Constant2/1 -> Product5/2
  Constant3/1 -> Product6/2
  Add/1 -> DenFek/1

== system modele_non_lineaire/ModeleNonLineaire/Simulation du système non-linéaire/Fa, Fb, Fc/Subsystem1/Subsystem2 ==
  I : Inport
  Abs : Abs
  Constant : Constant  Value=be1
  Product1 : Product
  Sign : Signum
  add 3 : Sum
  i1 : Product
  i2 : Product
  NumFek : Outport
  wires:
  i2/1 -> add 3/2
  Sign/1 -> Product1/2
  add 3/1 -> Product1/1
  Product1/1 -> NumFek/1
  I/1 -> Abs/1, i2/1, i2/2, Sign/1
  Constant/1 -> i1/1
  Abs/1 -> i1/2
  i1/1 -> add 3/1

== system modele_non_lineaire/ModeleNonLineaire/Simulation du système non-linéaire/Fa, Fb, Fc/Subsystem1/vtoi ==
  Vb : Inport
  Gain : Gain  Gain=1/LA
  Gain1 : Gain  Gain=RA/LA
  Integrator : Integrator  InitialCondition=ic_e
  Sum : Sum  Inputs=|+-
  i : Outport
  wires:
  Integrator/1 -> Gain1/1, i/1
  Gain/1 -> Sum/1
  Sum/1 -> Integrator/1
  Gain1/1 -> Sum/2
  Vb/1 -> Gain/1

== system modele_non_lineaire/ModeleNonLineaire/Simulation du système non-linéaire/Fa, Fb, Fc/Subsystem2/Subsystem ==
  z : Inport
  Add : Sum  Inputs=++++
  Constant : Constant  Value=as0
  Constant1 : Constant  Value=as1
  Constant2 : Constant  Value=as2
  Constant3 : Constant  Value=as3
  Product4 : Product
  Product5 : Product  Inputs=3
  Product6 : Product  Inputs=4
  DenFsk : Outport
  wires:
  Constant/1 -> Add/1
  Product5/1 -> Add/3
  Product4/1 -> Add/2
  Product6/1 -> Add/4
  z/1 -> Product5/3, Product6/1, Product6/4, Product6/3, Product5/1, Product4/1
  Constant1/1 -> Product4/2
  Constant2/1 -> Product5/2
  Constant3/1 -> Product6/2
  Add/1 -> DenFsk/1

== system modele_non_lineaire/ModeleNonLineaire/Simulation du système non-linéaire/Fa, Fb, Fc/Subsystem2/Subsystem1 ==
  z : Inport
  Add : Sum  Inputs=++++
  Constant : Constant  Value=ae0
  Constant1 : Constant  Value=ae1
  Constant2 : Constant  Value=ae2
  Constant3 : Constant  Value=ae3
  Product4 : Product
  Product5 : Product  Inputs=3
  Product6 : Product  Inputs=4
  DenFek : Outport
  wires:
  Constant/1 -> Add/1
  Product5/1 -> Add/3
  Product4/1 -> Add/2
  Product6/1 -> Add/4
  z/1 -> Product5/3, Product6/1, Product6/4, Product6/3, Product5/1, Product4/1
  Constant1/1 -> Product4/2
  Constant2/1 -> Product5/2
  Constant3/1 -> Product6/2
  Add/1 -> DenFek/1

== system modele_non_lineaire/ModeleNonLineaire/Simulation du système non-linéaire/Fa, Fb, Fc/Subsystem2/Subsystem2 ==
  I : Inport
  Abs : Abs
  Constant : Constant  Value=be1
  Product1 : Product
  Sign : Signum
  add 3 : Sum
  i1 : Product
  i2 : Product
  NumFek : Outport
  wires:
  i2/1 -> add 3/2
  Sign/1 -> Product1/2
  add 3/1 -> Product1/1
  Product1/1 -> NumFek/1
  I/1 -> Abs/1, i2/1, i2/2, Sign/1
  Constant/1 -> i1/1
  Abs/1 -> i1/2
  i1/1 -> add 3/1

== system modele_non_lineaire/ModeleNonLineaire/Simulation du système non-linéaire/Fa, Fb, Fc/Subsystem2/vtoi ==
  Vb : Inport
  Gain : Gain  Gain=1/LA
  Gain1 : Gain  Gain=RA/LA
  Integrator : Integrator  InitialCondition=ia_e
  Sum : Sum  Inputs=|+-
  i : Outport
  wires:
  Integrator/1 -> Gain1/1, i/1
  Gain/1 -> Sum/1
  Sum/1 -> Integrator/1
  Gain1/1 -> Sum/2
  Vb/1 -> Gain/1

== system modele_non_lineaire/ModeleNonLineaire/Simulation du système non-linéaire/Fa, Fb, Fc/Subsystem8/Subsystem ==
  z : Inport
  Add : Sum  Inputs=++++
  Constant : Constant  Value=as0
  Constant1 : Constant  Value=as1
  Constant2 : Constant  Value=as2
  Constant3 : Constant  Value=as3
  Product4 : Product
  Product5 : Product  Inputs=3
  Product6 : Product  Inputs=4
  DenFsk : Outport
  wires:
  Constant/1 -> Add/1
  Product5/1 -> Add/3
  Product4/1 -> Add/2
  Product6/1 -> Add/4
  z/1 -> Product6/1, Product6/4, Product6/3, Product5/3, Product5/1, Product4/1
  Constant1/1 -> Product4/2
  Constant2/1 -> Product5/2
  Constant3/1 -> Product6/2
  Add/1 -> DenFsk/1

== system modele_non_lineaire/ModeleNonLineaire/Simulation du système non-linéaire/Fa, Fb, Fc/Subsystem8/Subsystem1 ==
  z : Inport
  Add : Sum  Inputs=++++
  Constant : Constant  Value=ae0
  Constant1 : Constant  Value=ae1
  Constant2 : Constant  Value=ae2
  Constant3 : Constant  Value=ae3
  Product4 : Product
  Product5 : Product  Inputs=3
  Product6 : Product  Inputs=4
  DenFek : Outport
  wires:
  Constant/1 -> Add/1
  Product5/1 -> Add/3
  Product4/1 -> Add/2
  Product6/1 -> Add/4
  z/1 -> Product5/3, Product6/1, Product6/4, Product6/3, Product5/1, Product4/1
  Constant1/1 -> Product4/2
  Constant2/1 -> Product5/2
  Constant3/1 -> Product6/2
  Add/1 -> DenFek/1

== system modele_non_lineaire/ModeleNonLineaire/Simulation du système non-linéaire/Fa, Fb, Fc/Subsystem8/Subsystem2 ==
  I : Inport
  Abs : Abs
  Constant : Constant  Value=be1
  Product1 : Product
  Sign : Signum
  add 3 : Sum
  i1 : Product
  i2 : Product
  NumFek : Outport
  wires:
  i2/1 -> add 3/2
  Sign/1 -> Product1/2
  add 3/1 -> Product1/1
  Product1/1 -> NumFek/1
  I/1 -> Abs/1, i2/1, i2/2, Sign/1
  Constant/1 -> i1/1
  Abs/1 -> i1/2
  i1/1 -> add 3/1

== system modele_non_lineaire/ModeleNonLineaire/Simulation du système non-linéaire/Fa, Fb, Fc/Subsystem8/vtoi ==
  Vb : Inport
  Gain : Gain  Gain=1/LA
  Gain1 : Gain  Gain=RA/LA
  Integrator : Integrator  InitialCondition=ib_e
  Sum : Sum  Inputs=|+-
  i : Outport
  wires:
  Integrator/1 -> Gain1/1, i/1
  Gain/1 -> Sum/1
  Sum/1 -> Integrator/1
  Gain1/1 -> Sum/2
  Vb/1 -> Gain/1
